simulink model "V1"  (R2024a)
settings: Solver=VariableStepDiscrete  StartTime=0.0  StopTime=10.0  RelTol=1e-3
libraries: spsSeriesRLCBranchLib x7, spsCurrentMeasurementLib x6, spsMosfetLib x5, spsDCVoltageSourceLib x2, spsVoltageMeasurementLib x2, spsDiodeLib x1, eePwmGenerator x1, spsTriangleGeneratorLib x1, sps_lib x1
settings Model: Creator=MrEve  LastModifiedBy=MrEve

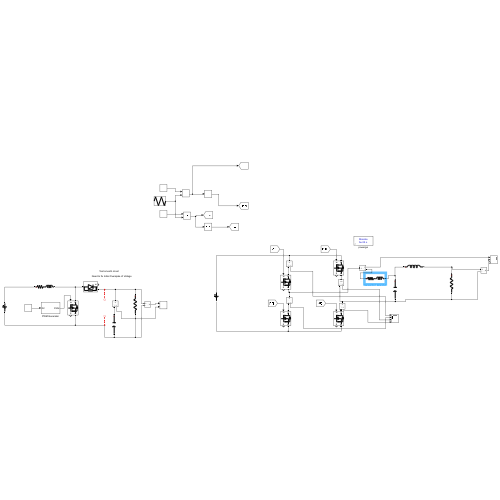
[thumbnail: Simulink's stored preview of the top-level diagram]
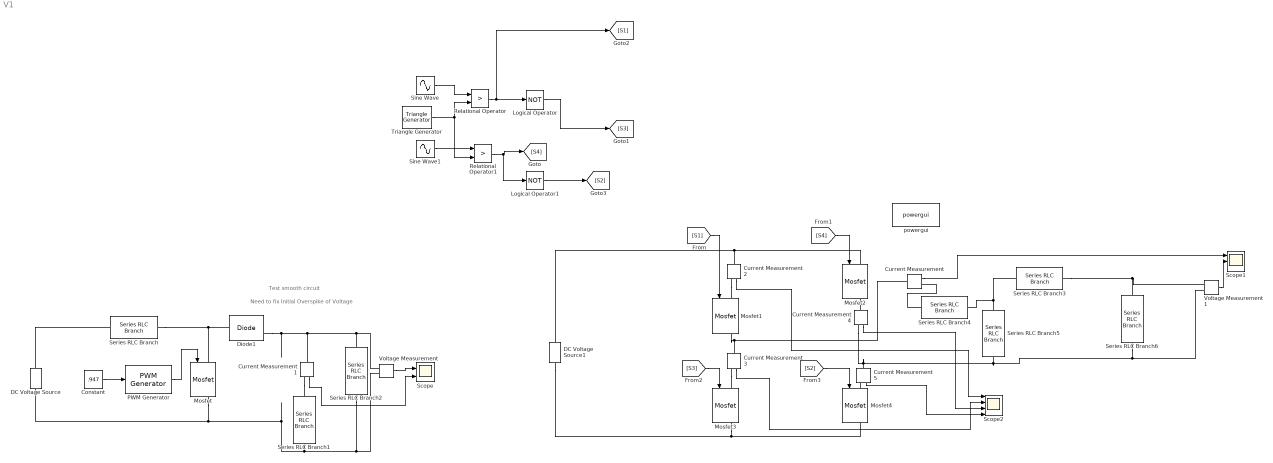
== system V1 ==
  note: Test smooth circuit
  note: Need to fix Initial Overspike of Voltage
  Constant : Constant  Value=.947
  Current Measurement{,1..5} (6 alike) : spsCurrentMeasurementLib/Current Measurement  PhasorSimulation=off  OutputType=Complex  PSBequivalent=0
  DC Voltage Source : spsDCVoltageSourceLib/DC Voltage Source  Amplitude=12  Measurements=None
  DC Voltage Source1 : spsDCVoltageSourceLib/DC Voltage Source  Amplitude=120  Measurements=None
  Diode1 : spsDiodeLib/Diode  Ron=0.001  Lon=0  Vf=0  IC=0  UseSnubber=0  Rs=3000  Cs=1e-6  Measurements=on
  Logical Operator : Logic  Operator=NOT  AllPortsSameDT=off  OutDataTypeStr=boolean
  Logical Operator1 : Logic  Operator=NOT  AllPortsSameDT=off  OutDataTypeStr=boolean
  Mosfet : spsMosfetLib/Mosfet  Ron=1e-3  Lon=0  Rd=1e-3  Vfd=0  IC=0  Rs=1e5  Cs=inf  Measurements=on
  Mosfet1 : spsMosfetLib/Mosfet  Ron=400e-3  Lon=0  Rd=1e-3  Vfd=0  IC=0  Rs=1e5  Cs=inf  Measurements=on
  Mosfet2 : spsMosfetLib/Mosfet  Ron=400e-03  Lon=0  Rd=1e-3  Vfd=0  IC=0  Rs=1e5  Cs=inf  Measurements=on
  Mosfet3 : spsMosfetLib/Mosfet  Ron=400e-3  Lon=0  Rd=1e-3  Vfd=0  IC=0  Rs=1e5  Cs=inf  Measurements=on
  Mosfet4 : spsMosfetLib/Mosfet  Ron=400e-3  Lon=0  Rd=1e-3  Vfd=0  IC=0  Rs=1e5  Cs=inf  Measurements=on
  PWM Generator : eePwmGenerator/PWM Generator  CarrCount=Up  Tper=0.001  Tdelay=0  Ts=5e-5
  Relational Operator : RelationalOperator  Operator=>  OutDataTypeStr=boolean  RndMeth=Simplest  InputSameDT=off
  Relational Operator1 : RelationalOperator  Operator=>  OutDataTypeStr=boolean  RndMeth=Simplest  InputSameDT=off
  Scope : Scope  NumInputPorts=2
  Scope1 : Scope  NumInputPorts=3
  Scope2 : Scope  NumInputPorts=4
  Series RLC Branch : spsSeriesRLCBranchLib/Series RLC Branch  LConnTagsString=__new0  RConnTagsString=__new0  BranchType=RL  Resistance=.001  Inductance=250e-6  SetiL0=off  InitialCurrent=0  Capacitance=1e-6  Setx0=off  InitialVoltage=0  Measurements=None
  Series RLC Branch1 : spsSeriesRLCBranchLib/Series RLC Branch  LConnTagsString=__new0  RConnTagsString=__new0  BranchType=C  Resistance=1  Inductance=1e-3  SetiL0=off  InitialCurrent=0  Capacitance=5000e-5  Setx0=off  InitialVoltage=0  Measurements=None
  Series RLC Branch2 : spsSeriesRLCBranchLib/Series RLC Branch  LConnTagsString=__new0  RConnTagsString=__new0  BranchType=R  Resistance=3  Inductance=1e-3  SetiL0=off  InitialCurrent=0  Capacitance=1e-6  Setx0=off  InitialVoltage=0  Measurements=None
  Series RLC Branch3 : spsSeriesRLCBranchLib/Series RLC Branch  LConnTagsString=__new0  RConnTagsString=__new0  BranchType=L  Resistance=1  Inductance=10e-3  SetiL0=off  InitialCurrent=0  Capacitance=10e-06  Setx0=off  InitialVoltage=0  Measurements=None
  Series RLC Branch4 : spsSeriesRLCBranchLib/Series RLC Branch  LConnTagsString=__new0  RConnTagsString=__new0  BranchType=RL  Resistance=900  Inductance=100e-3  SetiL0=off  InitialCurrent=0  Capacitance=10e-06  Setx0=off  InitialVoltage=0  Measurements=None
  Series RLC Branch5 : spsSeriesRLCBranchLib/Series RLC Branch  LConnTagsString=__new0  RConnTagsString=__new0  BranchType=C  Resistance=1  Inductance=2500e-6  SetiL0=off  InitialCurrent=0  Capacitance=1e-06  Setx0=off  InitialVoltage=0  Measurements=None
  Series RLC Branch6 : spsSeriesRLCBranchLib/Series RLC Branch  LConnTagsString=__new0  RConnTagsString=__new0  BranchType=R  Resistance=10000  Inductance=2500e-6  SetiL0=off  InitialCurrent=0  Capacitance=2e-06  Setx0=off  InitialVoltage=0  Measurements=None
  Sine Wave : Sin  Frequency=2*pi*60  SampleTime=0
  Sine Wave1 : Sin  Frequency=2*pi*60  Phase=pi  SampleTime=0
  Triangle Generator : spsTriangleGeneratorLib/Triangle Generator  Freq=1e3  Phase=90  Ts=0
  Voltage Measurement : spsVoltageMeasurementLib/Voltage Measurement  PhasorSimulation=off  OutputType=Complex  PSBequivalent=0
  Voltage Measurement1 : spsVoltageMeasurementLib/Voltage Measurement  PhasorSimulation=off  OutputType=Complex  PSBequivalent=0
  powergui : sps_lib/powergui  Priority=1  SimulationMode=Discrete  SampleTime=50e-6  frequency=60  Iterations=50  frequencyindice=0  Pbase=100e6  ErrMax=1e-4  UnitsV=kV  UnitsW=MW  buscounter=0  FunctionMessages=off  echomessages=off  EnableUseOfTLC=off  CurrentSourceSwitches=off  DisableSnubberDevices=off  DisableRonSwitches=off  DisableVfSwitches=off  DisplayEquations=off  AutomaticDiscreteSolvers=off  SolverType=Tustin/Backward Euler (TBE)  Interpol=off  ExternalGateDelay=off  methode=off  Ts=100  x0status=blocks  SPID=on  SwTol=0  HookPort=off  NonlinearTolerance=1e-4  nMaxIteration=100  ContinueOnMaxIteration=off  RestoreLinks=warning  ResistiveCurrentMeasurement=off  Frange=[0:2:500]  Ylog=off  Xlog=on  ShowGrid=off  save=off  variable=ZData  structure=0  ZoomFFT=off  StartTime=0.0  cycles=1  DisplayStyle=1  fundamental=60  FreqAxis=off  MaxFrequency=1000  frequencyindicesteady=1  RmsSteady=1  display=off
  wires:
  Sine Wave/1 -> Relational Operator/1
  Triangle Generator/1 -> Relational Operator/2, Relational Operator1/2
  Relational Operator/1 -> [S1], Logical Operator/1
  Logical Operator/1 -> [S3]
  [S1] -> Mosfet1/1
  [S4] -> Mosfet2/1
  [S2] -> Mosfet4/1
  [S3] -> Mosfet3/1
  Sine Wave1/1 -> Relational Operator1/1
  Relational Operator1/1 -> Logical Operator1/1, [S4]
  Logical Operator1/1 -> [S2]
  Voltage Measurement1/1 -> Scope1/2
  Constant/1 -> PWM Generator/1
  PWM Generator/1 -> Mosfet/1
  Voltage Measurement/1 -> Scope/1
  Current Measurement1/1 -> Scope/2
  Current Measurement/1 -> Scope1/1
  Current Measurement5/1 -> Scope2/4
  Current Measurement4/1 -> Scope2/3
  Current Measurement3/1 -> Scope2/2
  Current Measurement2/1 -> Scope2/1
  connections:
  DC Voltage Source1/RConn1 -- Current Measurement2/LConn1 -- Mosfet2/LConn1
  Mosfet3/RConn1 -- DC Voltage Source1/LConn1 -- Mosfet4/RConn1
  Mosfet1/RConn1 -- Current Measurement3/LConn1 -- Current Measurement/LConn1
  Series RLC Branch4/LConn1 -- Current Measurement/RConn1
  Series RLC Branch6/RConn1 -- Voltage Measurement1/LConn2 -- Current Measurement5/LConn1 -- Current Measurement4/RConn1 -- Series RLC Branch5/RConn1
  Diode1/RConn1 -- Series RLC Branch2/LConn1 -- Voltage Measurement/LConn1 -- Current Measurement1/LConn1
  Mosfet/LConn1 -- Diode1/LConn1 -- Series RLC Branch/RConn1
  Current Measurement1/RConn1 -- Series RLC Branch1/LConn1
  Series RLC Branch/LConn1 -- DC Voltage Source/RConn1
  DC Voltage Source/LConn1 -- Mosfet/RConn1 -- Voltage Measurement/LConn2 -- Series RLC Branch2/RConn1 -- Series RLC Branch1/RConn1
  Series RLC Branch4/RConn1 -- Series RLC Branch3/LConn1 -- Series RLC Branch5/LConn1
  Series RLC Branch3/RConn1 -- Series RLC Branch6/LConn1 -- Voltage Measurement1/LConn1
  Current Measurement2/RConn1 -- Mosfet1/LConn1
  Current Measurement3/RConn1 -- Mosfet3/LConn1
  Current Measurement4/LConn1 -- Mosfet2/RConn1
  Current Measurement5/RConn1 -- Mosfet4/LConn1
